simulink model "gm_Encoder_test"  (R2021b)
settings: Solver=FixedStepAuto  StartTime=0.0  StopTime=inf  RelTol=1e-3  EnableMultiTasking=on
libraries: simulink x2, hdlsllib x1
settings Model: Creator=Stijn  LastModifiedBy=Jeedella
settings SolverCC: AlgebraicLoopSolver=TrustRegion  PositivePriorityOrder=on
settings DataIOCC: ReturnWorkspaceOutputs=off
settings OptimizationCC: BlockReduction=off  ConditionallyExecuteInputs=off  DefaultParameterBehavior=Inlined  EnhancedBackFolding=on  PassReuseOutputArgsAs=Individual arguments  MaxStackSize=64  OptimizeBlockOrder=speed  DifferentSizesBufferReuse=on  OptimizationCustomize=off  EfficientTunableParamExpr=on
settings DebuggingCC: AlgebraicLoopMsg=error  InheritedTsInSrcMsg=none  ParameterTunabilityLossMsg=error  SFMachineParentedDataDiag=warning  ArithmeticOperatorsInVariantConditions=warning
settings HardwareCC: ProdBitPerPointer=32  ProdBitPerSizeT=32  ProdBitPerPtrDiffT=32  ProdLargestAtomicFloat=None  ProdIntDivRoundTo=Undefined  ProdEndianess=Unspecified  ProdWordSize=32  ProdHWDeviceType=ASIC/FPGA->ASIC/FPGA  TargetBitPerPointer=64  TargetBitPerSizeT=64  TargetBitPerPtrDiffT=64  TargetLongLongMode=on  TargetIntDivRoundTo=Zero  TargetEndianess=LittleEndian  TargetWordSize=64  TargetHWDeviceType=Custom Processor->MATLAB Host Computer  ProdEqTarget=off
settings SFSimCC: MATLABDynamicMemAlloc=off  CustomCodeUndefinedFunction=UseInterfaceOnly
settings RTWCC: Description=Embedded Coder  SystemTargetFile=ert.tlc  TemplateMakefile=ert_default_tmf  GenerateReport=on  Toolchain=Linaro AArch32 Linux v6.3.1  IncludeHyperlinkInReport=on  LaunchReport=on  GenerateTraceInfo=on  GenerateTraceReport=on  GenerateTraceReportSl=on  GenerateTraceReportSf=on  GenerateTraceReportEml=on
settings CodeAppCC: ForceParamTrailComments=on  IgnoreCustomStorageClasses=off  OperatorAnnotations=on  SimulinkDataObjDesc=on  SFDataObjDesc=on  InsertBlockDesc=on
settings ERTTargetCC: InlinedParameterPlacement=NonHierarchical  ERTCustomFileTemplate=example_file_process.tlc

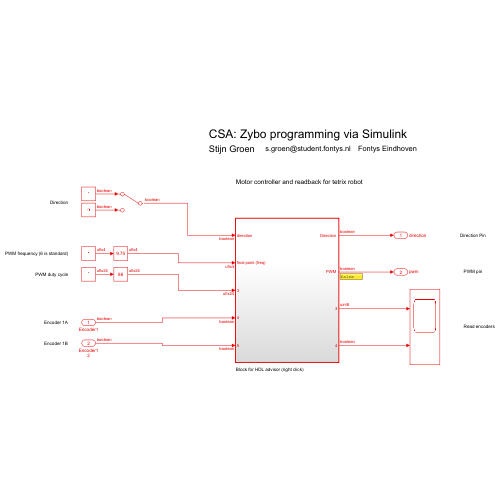
[thumbnail: Simulink's stored preview of the top-level diagram]
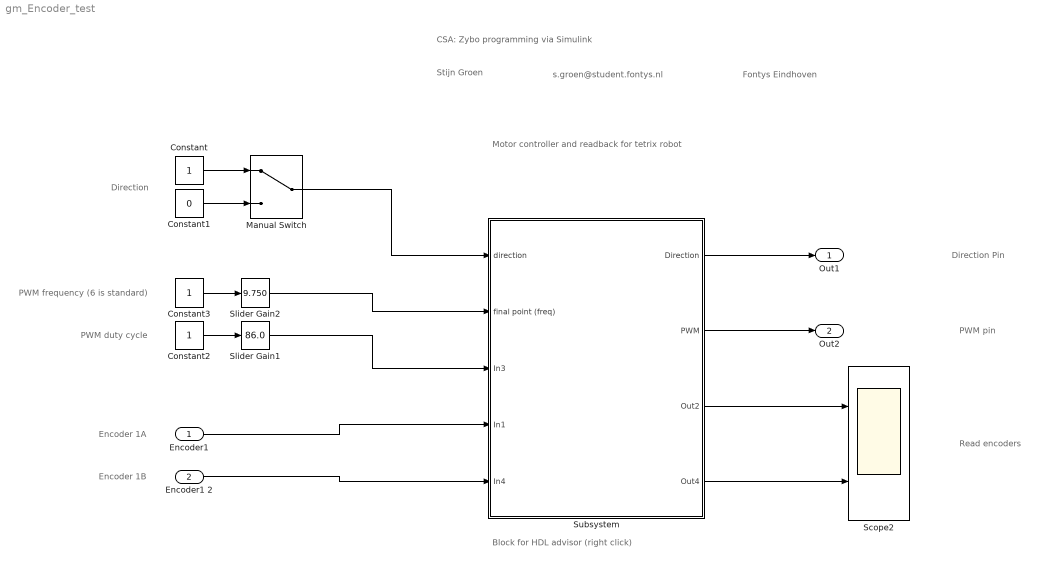
== system gm_Encoder_test ==
  note: CSA: Zybo programming via Simulink
  note: Stijn Groen
  note: s.groen@student.fontys.nl
  note: Fontys Eindhoven
  note: Block for HDL advisor (right click)
  note: Direction
  note: PWM frequency (6 is standard)
  note: PWM duty cycle
  note: Encoder 1A
  note: Encoder 1B
  note: Direction Pin
  note: PWM pin
  note: Read encoders
  note: Motor controller and readback for tetrix robot
  "Encoder1 " : Inport  OutDataTypeStr=boolean
  Encoder1 2 : Inport  Port=2  OutDataTypeStr=boolean
  Constant : Constant  OutDataTypeStr=boolean  SampleTime=-1
  Constant1 : Constant  Value=0  OutDataTypeStr=boolean  SampleTime=-1
  Constant2 : Constant  OutDataTypeStr=fixdt(0,24,0)  SampleTime=-1
  Constant3 : Constant  OutDataTypeStr=fixdt(0,4,0)  SampleTime=-1
  Manual Switch : ManualSwitch
  Scope2 : Scope  NumInputPorts=2
  Slider Gain1 : simulink/Math Operations/Slider Gain  gain=86.0  low=0  high=100
  Slider Gain2 : simulink/Math Operations/Slider Gain  gain=9.750  low=0  high=15
  Subsystem : Subsystem  TreatAsAtomicUnit=on
  Out1 : Outport  SignalName=direction  VectorParamsAs1DForOutWhenUnconnected=off
  Out2 : Outport  Port=2  SignalName=pwm  VectorParamsAs1DForOutWhenUnconnected=off
  wires:
  Subsystem/4(Out4) -> Scope2/2
  Encoder1 2/1 -> Subsystem/5(In4)
  "Encoder1 "/1 -> Subsystem/4(In1)
  Subsystem/3(Out2) -> Scope2/1
  Constant2/1 -> Slider Gain1/1
  Slider Gain1/1 -> Subsystem/3(In3)
  Slider Gain2/1 -> Subsystem/2("final point (freq) ")
  Subsystem/2("PWM ") -> Out2/1
  Subsystem/1("Direction ") -> Out1/1
  Manual Switch/1 -> Subsystem/1("direction ")
  Constant3/1 -> Slider Gain2/1
  Constant1/1 -> Manual Switch/2
  Constant/1 -> Manual Switch/1

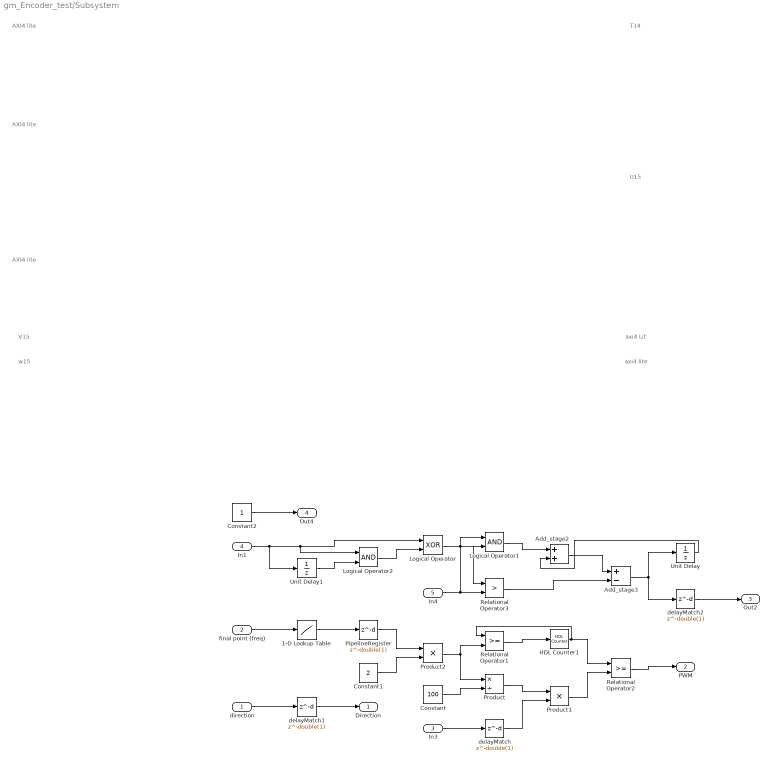
== system gm_Encoder_test/Subsystem ==
  note: AXI4 lite
  note: AXI4 lite
  note: AXI4 lite
  note: V15
  note: w15
  note: axi4 lite
  note: axi4 Lit
  note: U15
  note: T14
  "direction " : Inport  OutDataTypeStr=boolean  PortDimensions=1  SampleTime=0.0002
  "final point (freq) " : Inport  Port=2  OutDataTypeStr=fixdt(0, 4, 0)  PortDimensions=1  SampleTime=0.0002
  In3 : Inport  Port=3  OutDataTypeStr=fixdt(0, 24, 0)  PortDimensions=1  SampleTime=0.0002
  In1 : Inport  Port=4  OutDataTypeStr=boolean  PortDimensions=1  SampleTime=0.0002
  In4 : Inport  Port=5  OutDataTypeStr=boolean  PortDimensions=1  SampleTime=0.0002
  1-D Lookup Table : Lookup_n-D  NumberOfTableDimensions=1  BreakpointsSpecification=Even spacing  BreakpointsForDimension1=[1 2 3 4 5 6 7 8 9 10 11 12 13 14 15 16]  BreakpointsForDimension1FirstPoint=0  Table="reshape([8388607;4194304;2097152;1048576;524288;262144;131072;65536;32768;16384;8192;4096;2048;1024;512;256], [1  16])"  InterpMethod=Flat  DiagnosticForOutOfRangeInput=Error  OutDataTypeStr=fixdt(0, 24, 0)  RndMeth=Simplest  InputSameDT=on
  Add_stage2 : Sum  AccumDataTypeStr=uint8  OutDataTypeStr=uint8  SampleTime=0.0002
  Add_stage3 : Sum  Inputs=+-  AccumDataTypeStr=uint8  OutDataTypeStr=uint8  SampleTime=0.0002
  Constant : Constant  Value=100  OutDataTypeStr=fixdt(0, 24, 0)  SampleTime=-1
  Constant1 : Constant  Value=2  OutDataTypeStr=fixdt(0, 24, 0)  SampleTime=-1
  Constant2 : Constant  OutDataTypeStr=boolean  SampleTime=-1
  HDL Counter1 : hdlsllib/Sources/HDL Counter  CountType=Free running  CountInit=double(0)  CountStep=double(1)  CountMax=25  CountFromType=Initial value  CountFrom=double(0)  CountResetPort=on  CountLoadPort=off  CountEnbPort=off  CountDirPort=off  CountHitOutputPort=off  CountDataType=Unsigned  CountWordLen=24  CountFracLen=0  CountSampTime=0.0002
  Logical Operator : Logic  Operator=XOR  AllPortsSameDT=off  OutDataTypeStr=boolean  SampleTime=0.0002
  Logical Operator1 : Logic  AllPortsSameDT=off  OutDataTypeStr=boolean  SampleTime=0.0002
  Logical Operator2 : Logic  AllPortsSameDT=off  OutDataTypeStr=boolean  SampleTime=0.0002
  PipelineRegister : Delay  DelayLength=double(1)  InitialCondition=0  SampleTime=0.0002
  Product : Product  Inputs=*/  OutDataTypeStr=fixdt(0, 24, 0)  RndMeth=Simplest  SaturateOnIntegerOverflow=on  SampleTime=0.0002
  Product1 : Product  Inputs=**  OutDataTypeStr=fixdt(0, 24, 0)  RndMeth=Simplest  SampleTime=0.0002
  Product2 : Product  Inputs=**  OutDataTypeStr=fixdt(0, 24, 0)  RndMeth=Simplest  SampleTime=0.0002
  Relational Operator1 : RelationalOperator  OutDataTypeStr=boolean  SampleTime=0.0002  RndMeth=Nearest
  Relational Operator2 : RelationalOperator  OutDataTypeStr=boolean  SampleTime=0.0002  RndMeth=Nearest
  Relational Operator3 : RelationalOperator  Operator=>  OutDataTypeStr=boolean  SampleTime=0.0002  RndMeth=Nearest
  Unit Delay : UnitDelay  SampleTime=0.0002  HasFrameUpgradeWarning=on
  Unit Delay1 : UnitDelay  SampleTime=0.0002  HasFrameUpgradeWarning=on
  delayMatch : Delay  DelayLength=double(1)  InitialCondition=0  SampleTime=0.0002
  delayMatch1 : Delay  DelayLength=double(1)  InitialCondition=0  SampleTime=0.0002
  delayMatch2 : Delay  DelayLength=double(1)  InitialCondition=0  SampleTime=0.0002
  "Direction " : Outport  VectorParamsAs1DForOutWhenUnconnected=off
  "PWM " : Outport  Port=2  VectorParamsAs1DForOutWhenUnconnected=off
  Out2 : Outport  Port=3  VectorParamsAs1DForOutWhenUnconnected=off
  Out4 : Outport  Port=4  VectorParamsAs1DForOutWhenUnconnected=off
  wires:
  delayMatch1/1 -> "Direction "/1
  "final point (freq) "/1 -> 1-D Lookup Table/1
  delayMatch/1 -> Product1/2
  In1/1 -> Logical Operator2/1, Logical Operator/1, Unit Delay1/1
  In4/1 -> Relational Operator3/2, Logical Operator1/2
  PipelineRegister/1 -> Product2/1
  delayMatch2/1 -> Out2/1
  Constant/1 -> Product/2
  Constant1/1 -> Product2/2
  Constant2/1 -> Out4/1
  Logical Operator/1 -> Relational Operator3/1, Logical Operator1/1
  Logical Operator1/1 -> Add_stage2/1
  Logical Operator2/1 -> Logical Operator/2
  Product/1 -> Product1/1
  Product1/1 -> Relational Operator2/2
  Product2/1 -> Product/1, Relational Operator1/2
  Relational Operator2/1 -> "PWM "/1
  Relational Operator3/1 -> Add_stage3/2
  Unit Delay1/1 -> Logical Operator2/2
  In3/1 -> delayMatch/1
  "direction "/1 -> delayMatch1/1
  Add_stage3/1 -> delayMatch2/1, Unit Delay/1
  HDL Counter1/1 -> Relational Operator2/1, Relational Operator1/1
  Relational Operator1/1 -> HDL Counter1/1
  Unit Delay/1 -> Add_stage2/2
  Add_stage2/1 -> Add_stage3/1
  1-D Lookup Table/1 -> PipelineRegister/1
